simulink model "PD"  (R2013b)
settings: Solver=ode45  StartTime=0.0  StopTime=10.0  RelTol=1e-3
libraries: simulink x2
settings Model: Creator=USUARIO  LastModifiedBy=Usuario
settings DataIOCC: SignalLoggingSaveFormat=ModelDataLogs
settings DebuggingCC: UnderspecifiedInitializationDetection=Simplified  MultiTaskDSMMsg=warning  MultiTaskCondExecSysMsg=none
settings RTWCC: IncludeERTFirstTime=on
settings GRTTargetCC: CodeReplacementLibrary=None  CPPClassGenCompliant=on

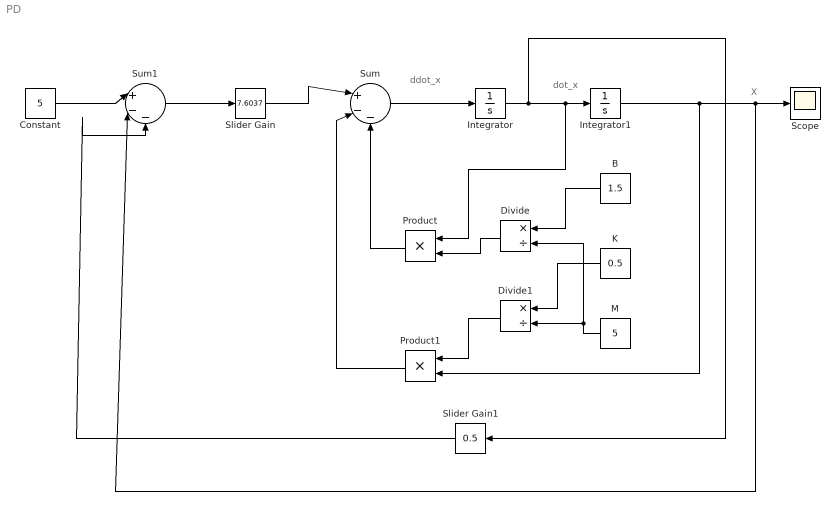
== system PD ==
  note: X
  note: dot_x
  note: ddot_x
  B : Constant  Value=1.5
  Constant : Constant  Value=5
  Divide : Product  Inputs=*/
  Divide1 : Product  Inputs=*/
  Integrator : Integrator
  Integrator1 : Integrator  InitialCondition=2
  K : Constant  Value=0.5
  M : Constant  Value=5
  Product : Product
  Product1 : Product
  Scope : Scope
  Slider Gain : simulink/Math Operations/Slider Gain  low=0  gain=7.6037  high=7.6037
  Slider Gain1 : simulink/Math Operations/Slider Gain  low=0  gain=0.5  high=7.6
  Sum : Sum  Inputs=|+--
  Sum1 : Sum  Inputs=|+--
  wires:
  Integrator/1 -> Integrator1/1, Product/1, Slider Gain1/1
  Sum/1 -> Integrator/1
  B/1 -> Divide/1
  M/1 -> Divide1/2, Divide/2
  K/1 -> Divide1/1
  Divide1/1 -> Product1/1
  Integrator1/1 -> Sum1/2, Scope/1, Product1/2
  Divide/1 -> Product/2
  Constant/1 -> Sum1/1
  Product/1 -> Sum/3
  Product1/1 -> Sum/2
  Slider Gain/1 -> Sum/1
  Sum1/1 -> Slider Gain/1
  Slider Gain1/1 -> Sum1/3
